simulink model "main_acs"  (R2025b)
settings: Solver=FixedStepAuto  StartTime=0.0  StopTime=20  FixedStep=0.001  RelTol=1e-3
values from neighbouring files (symbols this model uses):
  Actuator_MaxAngle = 8    [data.m]
  PID_Attitude_DCoeff_PY = 100    [data.m]
  PID_Attitude_DCoeff_R = 100    [data.m]
  PID_Attitude_Kd_PY = 0    [data.m]
  PID_Attitude_Kd_R = 0    [data.m]
  PID_Attitude_Ki_PY = 0    [data.m]
  PID_Attitude_Ki_R = 0    [data.m]
  PID_Attitude_Kp_PY = 2    [data.m]
  PID_Attitude_Kp_R = 2    [data.m]
  PID_Attitude_MaxOutput = 720    [data.m]
  PID_Attitude_SampleTime = 0.01    [data.m]
  PID_Guidance_K = 1/0.5    (= 2)    [data.m]
  PID_Guidance_MaxAcc = abs(5 * Physics_Gravity)    [data.m]
  PID_Guidance_N = 3.5    [data.m]
  PID_Guidance_SampleTime = 0.1    [data.m]
  PID_Rates_DCoeff_PY = 100    [data.m]
  PID_Rates_DCoeff_R = 100    [data.m]
  PID_Rates_Kd_PY = 0    [data.m]
  PID_Rates_Kd_R = 0    [data.m]
  PID_Rates_Ki_PY = 0    [data.m]
  PID_Rates_Ki_R = 0    [data.m]
  PID_Rates_Kp_PY = 400    [data.m]
  PID_Rates_Kp_R = 100    [data.m]
  PID_Rates_SampleTime = 0.002    [data.m]
libraries: slpidlib x6, simulink_extras x3, matrix_library x2, vrlib x1, aerolibanim x1
settings Model: Creator=Filip  LastModifiedBy=Filip
settings SolverCC: EnableFixedStepZeroCrossing=on
settings RTWCC: GenCodeOnly=on
settings SimscapeCC: SimscapeLogDecimation=1  SimscapeLogDataHistory=5000

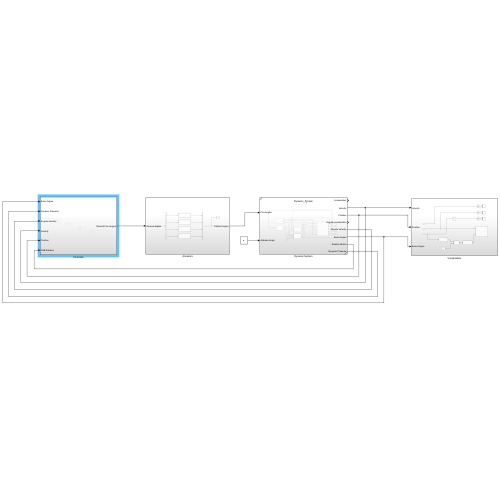
[thumbnail: Simulink's stored preview of the top-level diagram]
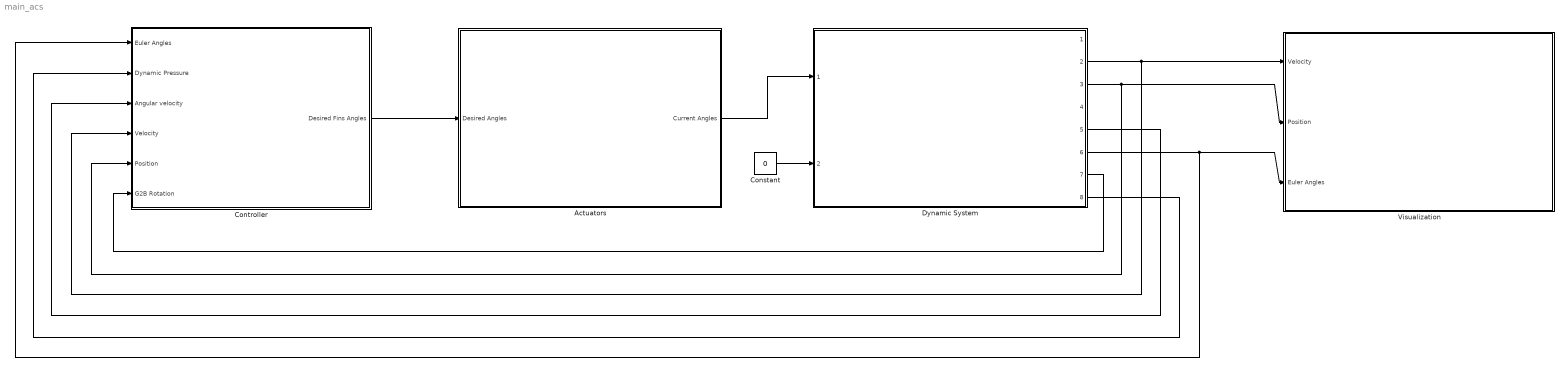
== system main_acs ==
  Actuators : Subsystem
  Constant : Constant  Value=0
  Controller : Subsystem
  Dynamic System : Subsystem  ReferencedSubsystem=Dynamic_System
  Visualization : Subsystem
  wires:
  Dynamic System/2 -> Controller/4(Velocity), Visualization/1(Velocity)
  Dynamic System/3 -> Controller/5(Position), Visualization/2(Position)
  Dynamic System/6 -> Controller/1(Euler Angles), Visualization/3(Euler Angles)
  Constant/1 -> Dynamic System/2
  Controller/1(Desired Fins Angles) -> Actuators/1(Desired Angles)
  Dynamic System/8 -> Controller/2(Dynamic Pressure)
  Dynamic System/5 -> Controller/3(Angular velocity)
  Dynamic System/7 -> Controller/6(G2B Rotation)
  Actuators/1(Current Angles) -> Dynamic System/1

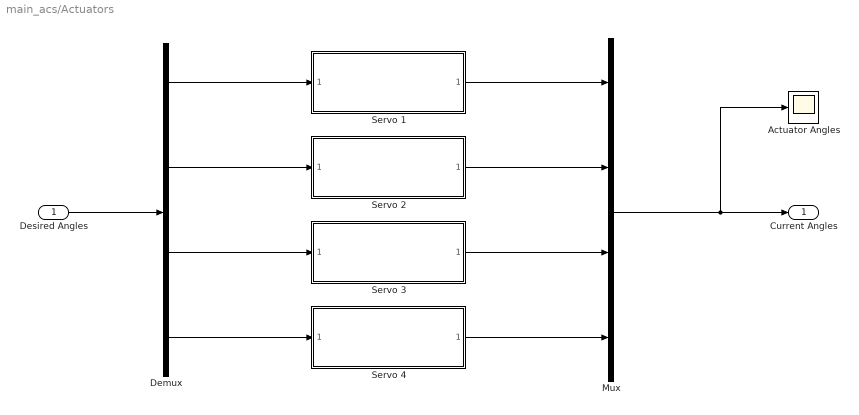
== system main_acs/Actuators ==
  Desired Angles : Inport
  Actuator Angles : Scope
      settings: ActiveDisplayYMinimum=-0.32568305206564774  ActiveDisplayYMaximum=0.47329758966714691  DataLoggingVariableName=ScopeData2
  Demux : Demux
  Mux : Mux
  Servo {1..4} (4 alike) : Subsystem  ReferencedSubsystem=Actuator_Dynamics
  Current Angles : Outport
  wires:
  Desired Angles/1 -> Demux/1
  Demux/1 -> Servo 1/1
  Demux/2 -> Servo 2/1
  Demux/3 -> Servo 3/1
  Demux/4 -> Servo 4/1
  Servo 1/1 -> Mux/1
  Servo 2/1 -> Mux/2
  Servo 3/1 -> Mux/3
  Servo 4/1 -> Mux/4
  Mux/1 -> Actuator Angles/1, Current Angles/1

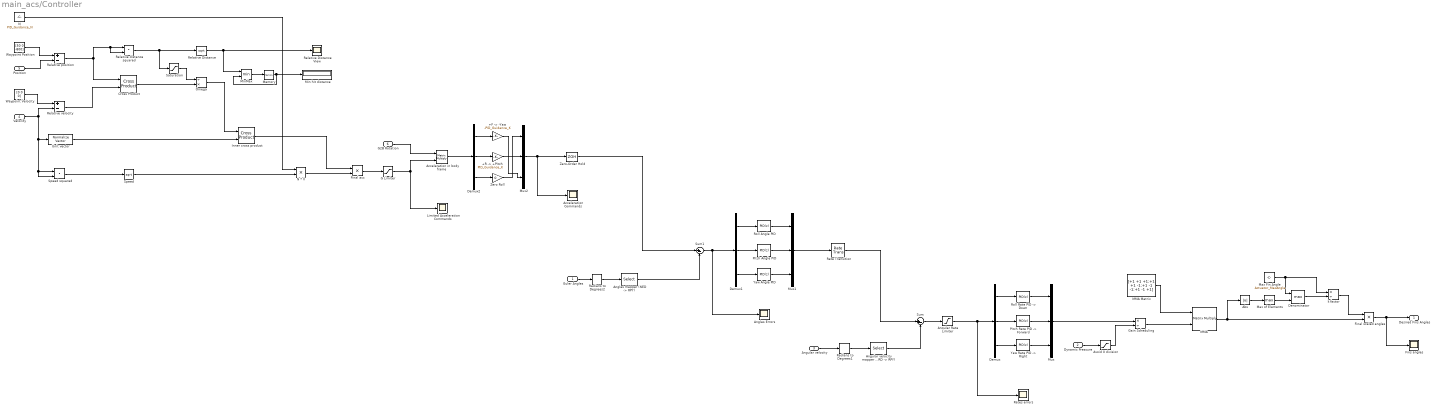
== system main_acs/Controller ==
  Euler Angles : Inport
  Dynamic Pressure : Inport  Port=2
  Angular velocity : Inport  Port=3
  Velocity : Inport  Port=4
  Position : Inport  Port=5
  G2B Rotation : Inport  Port=6
  "+F -> -Yaw" : Gain  Gain=-PID_Guidance_K
  "+R -> +Pitch" : Gain  Gain=PID_Guidance_K
  Abs : Abs  SaturateOnIntegerOverflow=off
  Acceleration Commands : Scope
      settings: ActiveDisplayYMinimum=-84.6659490201055  ActiveDisplayYMaximum=52.500724328147285  DataLoggingVariableName=ScopeData7
  Acceleration in body frame : Product  Multiplication=Matrix(*)
  Angles Errors : Scope
      settings: ActiveDisplayYMinimum=-272.55163687655789  ActiveDisplayYMaximum=253.11817045334493  DataLoggingVariableName=ScopeData6
  "Angles mapper (NED -> RPY)" : Selector  InputPortWidth=3  IndexOptions=Index vector (dialog)  Indices=[3 1 2]  OutputSizes=1
  Angular Rate Limiter : Saturate  UpperLimit=+PID_Attitude_MaxOutput  LowerLimit=-PID_Attitude_MaxOutput
  "Angular velocity mapper (FRD -> RPY)" : Selector  InputPortWidth=3  IndexOptions=Index vector (dialog)  Indices=[3 1 2]  OutputSizes=1
  Avoid 0 division : Saturate  UpperLimit=1000000  LowerLimit=10
  Cross Product : matrix_library/Cross Product
  Demux : Demux  Outputs=3
  Demux1 : Demux  Outputs=3
  Demux2 : Demux  Outputs=3
  Denominator : MinMax  Function=max  Inputs=2
  Final acc : Product
  Final scaled angles : Product
  Fins angles : Scope
      settings: ActiveDisplayYMinimum=-11.78731036094773  ActiveDisplayYMaximum=7.6919181875956841  DataLoggingVariableName=ScopeData5
  G Limiter : Saturate  UpperLimit=+PID_Guidance_MaxAcc  LowerLimit=-PID_Guidance_MaxAcc
  Gain Scheduling : Product  Inputs=*/
  Inner cross product : matrix_library/Cross Product
  Limited Acceleration Commands : Scope
      settings: ActiveDisplayYMinimum=-1  ActiveDisplayYMaximum=1  DataLoggingVariableName=ScopeData9
  MMA : Product  Multiplication=Matrix(*)
  MMA Matrix : Constant  Value=[+1 +1 +1;+1 +1 -1;+1 -1 -1;+1 -1 +1]
  Max Fin Angle : Constant  Value=Actuator_MaxAngle
  Max of Elements : MinMax  Function=max
  Memory : Memory  InitialCondition=inf
  Min hit distance : Display
  MinMax : MinMax  Inputs=2
  Mux : Mux  Inputs=3
  Mux1 : Mux  Inputs=3
  Mux2 : Mux  Inputs=3
  N : Constant  Value=PID_Guidance_N
  N * V : Product
  Omega : Product  Inputs=/*
  Pitch Angle PID : slpidlib/PID Controller  Controller=PID  Form=Parallel  TimeDomain=Discrete-time  UseExternalTs=off  SampleTime=PID_Attitude_SampleTime  IntegratorMethod=Forward Euler  FilterMethod=Forward Euler  ControllerParametersSource=internal  P=PID_Attitude_Kp_PY  I=PID_Attitude_Ki_PY  UseKiTs=off  D=PID_Attitude_Kd_PY  UseExternalDerivativeSource=off  N=PID_Attitude_DCoeff_PY  UseFilter=on  TunerSelectOption=Transfer Function Based (PID Tuner App)  InitialConditionSource=internal  InitialConditionForIntegrator=0  InitialConditionForFilter=0  DifferentiatorICPrevScaledInput=0  ExternalReset=none  TrackingMode=off  Kt=1  LimitOutput=off  SatLimitsSource=internal  UpperSaturationLimit=inf  LowerSaturationLimit=-inf  LinearizeAsGain=off  AntiWindupMode=back-calculation  Kb=1  LimitIntegrator=off  UpperIntegratorSaturationLimit=inf  LowerIntegratorSaturationLimit=-inf  POutMin=[]  POutMax=[]  IOutMin=[]  IOutMax=[]  DOutMin=[]  DOutMax=[]  NOutMin=[]  NOutMax=[]  SumOutMin=[]  SumOutMax=[]  SaturationOutMin=[]  SaturationOutMax=[]  PParamMin=[]  PParamMax=[]  IParamMin=[]  IParamMax=[]  DParamMin=[]  DParamMax=[]  NParamMin=[]  NParamMax=[]  KbParamMin=[]  KbParamMax=[]  KtParamMin=[]  KtParamMax=[]  KbOutMin=[]  KbOutMax=[]  KtOutMin=[]  KtOutMax=[]  IntegratorOutMin=[]  IntegratorOutMax=[]  FilterOutMin=[]  FilterOutMax=[]  SumI1OutMin=[]  SumI1OutMax=[]  SumI2OutMin=[]  SumI2OutMax=[]  SumI3OutMin=[]  SumI3OutMax=[]  SumI4OutMin=[]  SumI4OutMax=[]  SumDOutMin=[]  SumDOutMax=[]  DifferentiatorOutMin=[]  DifferentiatorOutMax=[]  FilterDiffOutCoefMin=[]  FilterDiffOutCoefMax=[]  ReciprocalOutMin=[]  ReciprocalOutMax=[]  SumDenOutMin=[]  SumDenOutMax=[]  SumNumOutMin=[]  SumNumOutMax=[]  DivideOutMin=[]  DivideOutMax=[]  UdiffTsProdOutMin=[]  UdiffTsProdOutMax=[]  NTsProdOutMin=[]  NTsProdOutMax=[]  UintegralTsProdOutMin=[]  UintegralTsProdOutMax=[]  UngainTsProdOutMin=[]  UngainTsProdOutMax=[]  ClampingZeroOutDataTypeStr=Inherit: Inherit via back propagation  ClampingZeroOutMin=[]  ClampingZeroOutMax=[]  FilterDenConstantOutDataTypeStr=Inherit: Inherit via back propagation  FilterDenConstantOutMin=[]  FilterDenConstantOutMax=[]  PCopyOutDataTypeStr=Inherit: Inherit via back propagation  PCopyOutMin=[]  PCopyOutMax=[]  NCopyOutDataTypeStr=Inherit: Inherit via back propagation  NCopyOutMin=[]  NCopyOutMax=[]  IntegratorContinuousStateAttributes=''  IntegratorStateMustResolveToSignalObject=off  IntegratorRTWStateStorageClass=Auto  FilterContinuousStateAttributes=''  FilterStateMustResolveToSignalObject=off  FilterRTWStateStorageClass=Auto  ParallelPVariant=InternalParameters  IdealPVariant=Disabled  IVariant=InternalParameters  DVariant=InternalParameters  IntegratorVariant=Discrete  SatVariant=Disabled  AWVariant=Passthrough  PCopyVariant=Disabled  TRVariant=Disabled  FdbkBlocksVariant=Forward  IdealPFdbkVariant=Disabled  SatFdbkVariant=Disabled  DerivativeFilterVariant=ForwardEulerFilter  NVariant=InternalParameters  NCopyVariant=Disabled  FilterICVariant=InternalICsFilter  IntegratorICVariant=InternalICs  ExternalResetVariant=Disabled  TRSumVariant=Passthrough  SumFdbkVariant=Disabled  SumVariant=Sum_PID  TsampFilterVariant=InternalTs  TsampNgainVariant=Passthrough  TsampIntegralVariant=Disabled_SignalSpec  ExternalSaturationOutDataTypeStr=Inherit: Same as second input  DerivativeSourceVariant=ErrorSignal  PreIntVariant=InternalPreInt
      settings: LibrarySourceBlock=simulink/Discrete/Discrete PID Controller
  "Pitch Rate PID -> Forward" : slpidlib/PID Controller  Controller=PID  Form=Parallel  TimeDomain=Discrete-time  UseExternalTs=off  SampleTime=PID_Rates_SampleTime  IntegratorMethod=Forward Euler  FilterMethod=Forward Euler  ControllerParametersSource=internal  P=PID_Rates_Kp_PY  I=PID_Rates_Ki_PY  UseKiTs=off  D=PID_Rates_Kd_PY  UseExternalDerivativeSource=off  N=PID_Rates_DCoeff_PY  UseFilter=on  TunerSelectOption=Transfer Function Based (PID Tuner App)  InitialConditionSource=internal  InitialConditionForIntegrator=0  InitialConditionForFilter=0  DifferentiatorICPrevScaledInput=0  ExternalReset=none  TrackingMode=off  Kt=1  LimitOutput=off  SatLimitsSource=internal  UpperSaturationLimit=inf  LowerSaturationLimit=-inf  LinearizeAsGain=off  AntiWindupMode=back-calculation  Kb=1  LimitIntegrator=off  UpperIntegratorSaturationLimit=inf  LowerIntegratorSaturationLimit=-inf  POutMin=[]  POutMax=[]  IOutMin=[]  IOutMax=[]  DOutMin=[]  DOutMax=[]  NOutMin=[]  NOutMax=[]  SumOutMin=[]  SumOutMax=[]  SaturationOutMin=[]  SaturationOutMax=[]  PParamMin=[]  PParamMax=[]  IParamMin=[]  IParamMax=[]  DParamMin=[]  DParamMax=[]  NParamMin=[]  NParamMax=[]  KbParamMin=[]  KbParamMax=[]  KtParamMin=[]  KtParamMax=[]  KbOutMin=[]  KbOutMax=[]  KtOutMin=[]  KtOutMax=[]  IntegratorOutMin=[]  IntegratorOutMax=[]  FilterOutMin=[]  FilterOutMax=[]  SumI1OutMin=[]  SumI1OutMax=[]  SumI2OutMin=[]  SumI2OutMax=[]  SumI3OutMin=[]  SumI3OutMax=[]  SumI4OutMin=[]  SumI4OutMax=[]  SumDOutMin=[]  SumDOutMax=[]  DifferentiatorOutMin=[]  DifferentiatorOutMax=[]  FilterDiffOutCoefMin=[]  FilterDiffOutCoefMax=[]  ReciprocalOutMin=[]  ReciprocalOutMax=[]  SumDenOutMin=[]  SumDenOutMax=[]  SumNumOutMin=[]  SumNumOutMax=[]  DivideOutMin=[]  DivideOutMax=[]  UdiffTsProdOutMin=[]  UdiffTsProdOutMax=[]  NTsProdOutMin=[]  NTsProdOutMax=[]  UintegralTsProdOutMin=[]  UintegralTsProdOutMax=[]  UngainTsProdOutMin=[]  UngainTsProdOutMax=[]  ClampingZeroOutDataTypeStr=Inherit: Inherit via back propagation  ClampingZeroOutMin=[]  ClampingZeroOutMax=[]  FilterDenConstantOutDataTypeStr=Inherit: Inherit via back propagation  FilterDenConstantOutMin=[]  FilterDenConstantOutMax=[]  PCopyOutDataTypeStr=Inherit: Inherit via back propagation  PCopyOutMin=[]  PCopyOutMax=[]  NCopyOutDataTypeStr=Inherit: Inherit via back propagation  NCopyOutMin=[]  NCopyOutMax=[]  IntegratorContinuousStateAttributes=''  IntegratorStateMustResolveToSignalObject=off  IntegratorRTWStateStorageClass=Auto  FilterContinuousStateAttributes=''  FilterStateMustResolveToSignalObject=off  FilterRTWStateStorageClass=Auto  ParallelPVariant=InternalParameters  IdealPVariant=Disabled  IVariant=InternalParameters  DVariant=InternalParameters  IntegratorVariant=Discrete  SatVariant=Disabled  AWVariant=Passthrough  PCopyVariant=Disabled  TRVariant=Disabled  FdbkBlocksVariant=Forward  IdealPFdbkVariant=Disabled  SatFdbkVariant=Disabled  DerivativeFilterVariant=ForwardEulerFilter  NVariant=InternalParameters  NCopyVariant=Disabled  FilterICVariant=InternalICsFilter  IntegratorICVariant=InternalICs  ExternalResetVariant=Disabled  TRSumVariant=Passthrough  SumFdbkVariant=Disabled  SumVariant=Sum_PID  TsampFilterVariant=InternalTs  TsampNgainVariant=Passthrough  TsampIntegralVariant=Disabled_SignalSpec  ExternalSaturationOutDataTypeStr=Inherit: Same as second input  DerivativeSourceVariant=ErrorSignal  PreIntVariant=InternalPreInt
      settings: LibrarySourceBlock=simulink/Discrete/Discrete PID Controller
  Radians to Degrees1 : simulink_extras/Transformations/Radians to Degrees
  Radians to Degrees2 : simulink_extras/Transformations/Radians to Degrees
  Rate Transition : RateTransition
  Rates errors : Scope
      settings: ActiveDisplayYMinimum=-72.348500996231849  ActiveDisplayYMaximum=106.71571719199865  DataLoggingVariableName=ScopeData4
  Relative Distance : Sqrt
  Relative Distance View : Scope
      settings: ActiveDisplayYMinimum=-3326.7909111536519  ActiveDisplayYMaximum=1807.9538182461531  DataLoggingVariableName=ScopeData8
  Relative distance squared : DotProduct  OutDataTypeStr=Inherit: Inherit via internal rule
  Relative position : Sum  Inputs=+-
  Relative velocity : Sum  Inputs=+-
  Roll Angle PID : slpidlib/PID Controller  Controller=PID  Form=Parallel  TimeDomain=Discrete-time  UseExternalTs=off  SampleTime=PID_Attitude_SampleTime  IntegratorMethod=Forward Euler  FilterMethod=Forward Euler  ControllerParametersSource=internal  P=PID_Attitude_Kp_R  I=PID_Attitude_Ki_R  UseKiTs=off  D=PID_Attitude_Kd_R  UseExternalDerivativeSource=off  N=PID_Attitude_DCoeff_R  UseFilter=on  TunerSelectOption=Transfer Function Based (PID Tuner App)  InitialConditionSource=internal  InitialConditionForIntegrator=0  InitialConditionForFilter=0  DifferentiatorICPrevScaledInput=0  ExternalReset=none  TrackingMode=off  Kt=1  LimitOutput=off  SatLimitsSource=internal  UpperSaturationLimit=inf  LowerSaturationLimit=-inf  LinearizeAsGain=off  AntiWindupMode=back-calculation  Kb=1  LimitIntegrator=off  UpperIntegratorSaturationLimit=inf  LowerIntegratorSaturationLimit=-inf  POutMin=[]  POutMax=[]  IOutMin=[]  IOutMax=[]  DOutMin=[]  DOutMax=[]  NOutMin=[]  NOutMax=[]  SumOutMin=[]  SumOutMax=[]  SaturationOutMin=[]  SaturationOutMax=[]  PParamMin=[]  PParamMax=[]  IParamMin=[]  IParamMax=[]  DParamMin=[]  DParamMax=[]  NParamMin=[]  NParamMax=[]  KbParamMin=[]  KbParamMax=[]  KtParamMin=[]  KtParamMax=[]  KbOutMin=[]  KbOutMax=[]  KtOutMin=[]  KtOutMax=[]  IntegratorOutMin=[]  IntegratorOutMax=[]  FilterOutMin=[]  FilterOutMax=[]  SumI1OutMin=[]  SumI1OutMax=[]  SumI2OutMin=[]  SumI2OutMax=[]  SumI3OutMin=[]  SumI3OutMax=[]  SumI4OutMin=[]  SumI4OutMax=[]  SumDOutMin=[]  SumDOutMax=[]  DifferentiatorOutMin=[]  DifferentiatorOutMax=[]  FilterDiffOutCoefMin=[]  FilterDiffOutCoefMax=[]  ReciprocalOutMin=[]  ReciprocalOutMax=[]  SumDenOutMin=[]  SumDenOutMax=[]  SumNumOutMin=[]  SumNumOutMax=[]  DivideOutMin=[]  DivideOutMax=[]  UdiffTsProdOutMin=[]  UdiffTsProdOutMax=[]  NTsProdOutMin=[]  NTsProdOutMax=[]  UintegralTsProdOutMin=[]  UintegralTsProdOutMax=[]  UngainTsProdOutMin=[]  UngainTsProdOutMax=[]  ClampingZeroOutDataTypeStr=Inherit: Inherit via back propagation  ClampingZeroOutMin=[]  ClampingZeroOutMax=[]  FilterDenConstantOutDataTypeStr=Inherit: Inherit via back propagation  FilterDenConstantOutMin=[]  FilterDenConstantOutMax=[]  PCopyOutDataTypeStr=Inherit: Inherit via back propagation  PCopyOutMin=[]  PCopyOutMax=[]  NCopyOutDataTypeStr=Inherit: Inherit via back propagation  NCopyOutMin=[]  NCopyOutMax=[]  IntegratorContinuousStateAttributes=''  IntegratorStateMustResolveToSignalObject=off  IntegratorRTWStateStorageClass=Auto  FilterContinuousStateAttributes=''  FilterStateMustResolveToSignalObject=off  FilterRTWStateStorageClass=Auto  ParallelPVariant=InternalParameters  IdealPVariant=Disabled  IVariant=InternalParameters  DVariant=InternalParameters  IntegratorVariant=Discrete  SatVariant=Disabled  AWVariant=Passthrough  PCopyVariant=Disabled  TRVariant=Disabled  FdbkBlocksVariant=Forward  IdealPFdbkVariant=Disabled  SatFdbkVariant=Disabled  DerivativeFilterVariant=ForwardEulerFilter  NVariant=InternalParameters  NCopyVariant=Disabled  FilterICVariant=InternalICsFilter  IntegratorICVariant=InternalICs  ExternalResetVariant=Disabled  TRSumVariant=Passthrough  SumFdbkVariant=Disabled  SumVariant=Sum_PID  TsampFilterVariant=InternalTs  TsampNgainVariant=Passthrough  TsampIntegralVariant=Disabled_SignalSpec  ExternalSaturationOutDataTypeStr=Inherit: Same as second input  DerivativeSourceVariant=ErrorSignal  PreIntVariant=InternalPreInt
      settings: LibrarySourceBlock=simulink/Discrete/Discrete PID Controller
  "Roll Rate PID -> Down" : slpidlib/PID Controller  Controller=PID  Form=Parallel  TimeDomain=Discrete-time  UseExternalTs=off  SampleTime=PID_Rates_SampleTime  IntegratorMethod=Forward Euler  FilterMethod=Forward Euler  ControllerParametersSource=internal  P=PID_Rates_Kp_R  I=PID_Rates_Ki_R  UseKiTs=off  D=PID_Rates_Kd_R  UseExternalDerivativeSource=off  N=PID_Rates_DCoeff_R  UseFilter=on  TunerSelectOption=Transfer Function Based (PID Tuner App)  InitialConditionSource=internal  InitialConditionForIntegrator=0  InitialConditionForFilter=0  DifferentiatorICPrevScaledInput=0  ExternalReset=none  TrackingMode=off  Kt=1  LimitOutput=off  SatLimitsSource=internal  UpperSaturationLimit=inf  LowerSaturationLimit=-inf  LinearizeAsGain=off  AntiWindupMode=back-calculation  Kb=1  LimitIntegrator=off  UpperIntegratorSaturationLimit=inf  LowerIntegratorSaturationLimit=-inf  POutMin=[]  POutMax=[]  IOutMin=[]  IOutMax=[]  DOutMin=[]  DOutMax=[]  NOutMin=[]  NOutMax=[]  SumOutMin=[]  SumOutMax=[]  SaturationOutMin=[]  SaturationOutMax=[]  PParamMin=[]  PParamMax=[]  IParamMin=[]  IParamMax=[]  DParamMin=[]  DParamMax=[]  NParamMin=[]  NParamMax=[]  KbParamMin=[]  KbParamMax=[]  KtParamMin=[]  KtParamMax=[]  KbOutMin=[]  KbOutMax=[]  KtOutMin=[]  KtOutMax=[]  IntegratorOutMin=[]  IntegratorOutMax=[]  FilterOutMin=[]  FilterOutMax=[]  SumI1OutMin=[]  SumI1OutMax=[]  SumI2OutMin=[]  SumI2OutMax=[]  SumI3OutMin=[]  SumI3OutMax=[]  SumI4OutMin=[]  SumI4OutMax=[]  SumDOutMin=[]  SumDOutMax=[]  DifferentiatorOutMin=[]  DifferentiatorOutMax=[]  FilterDiffOutCoefMin=[]  FilterDiffOutCoefMax=[]  ReciprocalOutMin=[]  ReciprocalOutMax=[]  SumDenOutMin=[]  SumDenOutMax=[]  SumNumOutMin=[]  SumNumOutMax=[]  DivideOutMin=[]  DivideOutMax=[]  UdiffTsProdOutMin=[]  UdiffTsProdOutMax=[]  NTsProdOutMin=[]  NTsProdOutMax=[]  UintegralTsProdOutMin=[]  UintegralTsProdOutMax=[]  UngainTsProdOutMin=[]  UngainTsProdOutMax=[]  ClampingZeroOutDataTypeStr=Inherit: Inherit via back propagation  ClampingZeroOutMin=[]  ClampingZeroOutMax=[]  FilterDenConstantOutDataTypeStr=Inherit: Inherit via back propagation  FilterDenConstantOutMin=[]  FilterDenConstantOutMax=[]  PCopyOutDataTypeStr=Inherit: Inherit via back propagation  PCopyOutMin=[]  PCopyOutMax=[]  NCopyOutDataTypeStr=Inherit: Inherit via back propagation  NCopyOutMin=[]  NCopyOutMax=[]  IntegratorContinuousStateAttributes=''  IntegratorStateMustResolveToSignalObject=off  IntegratorRTWStateStorageClass=Auto  FilterContinuousStateAttributes=''  FilterStateMustResolveToSignalObject=off  FilterRTWStateStorageClass=Auto  ParallelPVariant=InternalParameters  IdealPVariant=Disabled  IVariant=InternalParameters  DVariant=InternalParameters  IntegratorVariant=Discrete  SatVariant=Disabled  AWVariant=Passthrough  PCopyVariant=Disabled  TRVariant=Disabled  FdbkBlocksVariant=Forward  IdealPFdbkVariant=Disabled  SatFdbkVariant=Disabled  DerivativeFilterVariant=ForwardEulerFilter  NVariant=InternalParameters  NCopyVariant=Disabled  FilterICVariant=InternalICsFilter  IntegratorICVariant=InternalICs  ExternalResetVariant=Disabled  TRSumVariant=Passthrough  SumFdbkVariant=Disabled  SumVariant=Sum_PID  TsampFilterVariant=InternalTs  TsampNgainVariant=Passthrough  TsampIntegralVariant=Disabled_SignalSpec  ExternalSaturationOutDataTypeStr=Inherit: Same as second input  DerivativeSourceVariant=ErrorSignal  PreIntVariant=InternalPreInt
      settings: LibrarySourceBlock=simulink/Discrete/Discrete PID Controller
  Saturation : Saturate  UpperLimit=10000000  LowerLimit=400
  Speed : Sqrt
  Speed squared : DotProduct  OutDataTypeStr=Inherit: Inherit via internal rule
  Sum : Sum  Inputs=|+-
  Sum1 : Sum  Inputs=|+-
  Unit vector : vrlib/Utilities/Normalize Vector  maxzero=0
  Waypoint Position : Constant  Value=[50 0 -800]
  Waypoint Velocity : Constant  Value=[0 0 0]
  Yaw Angle PID : slpidlib/PID Controller  Controller=PID  Form=Parallel  TimeDomain=Discrete-time  UseExternalTs=off  SampleTime=PID_Attitude_SampleTime  IntegratorMethod=Forward Euler  FilterMethod=Forward Euler  ControllerParametersSource=internal  P=PID_Attitude_Kp_PY  I=PID_Attitude_Ki_PY  UseKiTs=off  D=PID_Attitude_Kd_PY  UseExternalDerivativeSource=off  N=PID_Attitude_DCoeff_PY  UseFilter=on  TunerSelectOption=Transfer Function Based (PID Tuner App)  InitialConditionSource=internal  InitialConditionForIntegrator=0  InitialConditionForFilter=0  DifferentiatorICPrevScaledInput=0  ExternalReset=none  TrackingMode=off  Kt=1  LimitOutput=off  SatLimitsSource=internal  UpperSaturationLimit=inf  LowerSaturationLimit=-inf  LinearizeAsGain=off  AntiWindupMode=back-calculation  Kb=1  LimitIntegrator=off  UpperIntegratorSaturationLimit=inf  LowerIntegratorSaturationLimit=-inf  POutMin=[]  POutMax=[]  IOutMin=[]  IOutMax=[]  DOutMin=[]  DOutMax=[]  NOutMin=[]  NOutMax=[]  SumOutMin=[]  SumOutMax=[]  SaturationOutMin=[]  SaturationOutMax=[]  PParamMin=[]  PParamMax=[]  IParamMin=[]  IParamMax=[]  DParamMin=[]  DParamMax=[]  NParamMin=[]  NParamMax=[]  KbParamMin=[]  KbParamMax=[]  KtParamMin=[]  KtParamMax=[]  KbOutMin=[]  KbOutMax=[]  KtOutMin=[]  KtOutMax=[]  IntegratorOutMin=[]  IntegratorOutMax=[]  FilterOutMin=[]  FilterOutMax=[]  SumI1OutMin=[]  SumI1OutMax=[]  SumI2OutMin=[]  SumI2OutMax=[]  SumI3OutMin=[]  SumI3OutMax=[]  SumI4OutMin=[]  SumI4OutMax=[]  SumDOutMin=[]  SumDOutMax=[]  DifferentiatorOutMin=[]  DifferentiatorOutMax=[]  FilterDiffOutCoefMin=[]  FilterDiffOutCoefMax=[]  ReciprocalOutMin=[]  ReciprocalOutMax=[]  SumDenOutMin=[]  SumDenOutMax=[]  SumNumOutMin=[]  SumNumOutMax=[]  DivideOutMin=[]  DivideOutMax=[]  UdiffTsProdOutMin=[]  UdiffTsProdOutMax=[]  NTsProdOutMin=[]  NTsProdOutMax=[]  UintegralTsProdOutMin=[]  UintegralTsProdOutMax=[]  UngainTsProdOutMin=[]  UngainTsProdOutMax=[]  ClampingZeroOutDataTypeStr=Inherit: Inherit via back propagation  ClampingZeroOutMin=[]  ClampingZeroOutMax=[]  FilterDenConstantOutDataTypeStr=Inherit: Inherit via back propagation  FilterDenConstantOutMin=[]  FilterDenConstantOutMax=[]  PCopyOutDataTypeStr=Inherit: Inherit via back propagation  PCopyOutMin=[]  PCopyOutMax=[]  NCopyOutDataTypeStr=Inherit: Inherit via back propagation  NCopyOutMin=[]  NCopyOutMax=[]  IntegratorContinuousStateAttributes=''  IntegratorStateMustResolveToSignalObject=off  IntegratorRTWStateStorageClass=Auto  FilterContinuousStateAttributes=''  FilterStateMustResolveToSignalObject=off  FilterRTWStateStorageClass=Auto  ParallelPVariant=InternalParameters  IdealPVariant=Disabled  IVariant=InternalParameters  DVariant=InternalParameters  IntegratorVariant=Discrete  SatVariant=Disabled  AWVariant=Passthrough  PCopyVariant=Disabled  TRVariant=Disabled  FdbkBlocksVariant=Forward  IdealPFdbkVariant=Disabled  SatFdbkVariant=Disabled  DerivativeFilterVariant=ForwardEulerFilter  NVariant=InternalParameters  NCopyVariant=Disabled  FilterICVariant=InternalICsFilter  IntegratorICVariant=InternalICs  ExternalResetVariant=Disabled  TRSumVariant=Passthrough  SumFdbkVariant=Disabled  SumVariant=Sum_PID  TsampFilterVariant=InternalTs  TsampNgainVariant=Passthrough  TsampIntegralVariant=Disabled_SignalSpec  ExternalSaturationOutDataTypeStr=Inherit: Same as second input  DerivativeSourceVariant=ErrorSignal  PreIntVariant=InternalPreInt
      settings: LibrarySourceBlock=simulink/Discrete/Discrete PID Controller
  "Yaw Rate PID -> Right" : slpidlib/PID Controller  Controller=PID  Form=Parallel  TimeDomain=Discrete-time  UseExternalTs=off  SampleTime=PID_Rates_SampleTime  IntegratorMethod=Forward Euler  FilterMethod=Forward Euler  ControllerParametersSource=internal  P=PID_Rates_Kp_PY  I=PID_Rates_Ki_PY  UseKiTs=off  D=PID_Rates_Kd_PY  UseExternalDerivativeSource=off  N=PID_Rates_DCoeff_PY  UseFilter=on  TunerSelectOption=Transfer Function Based (PID Tuner App)  InitialConditionSource=internal  InitialConditionForIntegrator=0  InitialConditionForFilter=0  DifferentiatorICPrevScaledInput=0  ExternalReset=none  TrackingMode=off  Kt=1  LimitOutput=off  SatLimitsSource=internal  UpperSaturationLimit=inf  LowerSaturationLimit=-inf  LinearizeAsGain=off  AntiWindupMode=back-calculation  Kb=1  LimitIntegrator=off  UpperIntegratorSaturationLimit=inf  LowerIntegratorSaturationLimit=-inf  POutMin=[]  POutMax=[]  IOutMin=[]  IOutMax=[]  DOutMin=[]  DOutMax=[]  NOutMin=[]  NOutMax=[]  SumOutMin=[]  SumOutMax=[]  SaturationOutMin=[]  SaturationOutMax=[]  PParamMin=[]  PParamMax=[]  IParamMin=[]  IParamMax=[]  DParamMin=[]  DParamMax=[]  NParamMin=[]  NParamMax=[]  KbParamMin=[]  KbParamMax=[]  KtParamMin=[]  KtParamMax=[]  KbOutMin=[]  KbOutMax=[]  KtOutMin=[]  KtOutMax=[]  IntegratorOutMin=[]  IntegratorOutMax=[]  FilterOutMin=[]  FilterOutMax=[]  SumI1OutMin=[]  SumI1OutMax=[]  SumI2OutMin=[]  SumI2OutMax=[]  SumI3OutMin=[]  SumI3OutMax=[]  SumI4OutMin=[]  SumI4OutMax=[]  SumDOutMin=[]  SumDOutMax=[]  DifferentiatorOutMin=[]  DifferentiatorOutMax=[]  FilterDiffOutCoefMin=[]  FilterDiffOutCoefMax=[]  ReciprocalOutMin=[]  ReciprocalOutMax=[]  SumDenOutMin=[]  SumDenOutMax=[]  SumNumOutMin=[]  SumNumOutMax=[]  DivideOutMin=[]  DivideOutMax=[]  UdiffTsProdOutMin=[]  UdiffTsProdOutMax=[]  NTsProdOutMin=[]  NTsProdOutMax=[]  UintegralTsProdOutMin=[]  UintegralTsProdOutMax=[]  UngainTsProdOutMin=[]  UngainTsProdOutMax=[]  ClampingZeroOutDataTypeStr=Inherit: Inherit via back propagation  ClampingZeroOutMin=[]  ClampingZeroOutMax=[]  FilterDenConstantOutDataTypeStr=Inherit: Inherit via back propagation  FilterDenConstantOutMin=[]  FilterDenConstantOutMax=[]  PCopyOutDataTypeStr=Inherit: Inherit via back propagation  PCopyOutMin=[]  PCopyOutMax=[]  NCopyOutDataTypeStr=Inherit: Inherit via back propagation  NCopyOutMin=[]  NCopyOutMax=[]  IntegratorContinuousStateAttributes=''  IntegratorStateMustResolveToSignalObject=off  IntegratorRTWStateStorageClass=Auto  FilterContinuousStateAttributes=''  FilterStateMustResolveToSignalObject=off  FilterRTWStateStorageClass=Auto  ParallelPVariant=InternalParameters  IdealPVariant=Disabled  IVariant=InternalParameters  DVariant=InternalParameters  IntegratorVariant=Discrete  SatVariant=Disabled  AWVariant=Passthrough  PCopyVariant=Disabled  TRVariant=Disabled  FdbkBlocksVariant=Forward  IdealPFdbkVariant=Disabled  SatFdbkVariant=Disabled  DerivativeFilterVariant=ForwardEulerFilter  NVariant=InternalParameters  NCopyVariant=Disabled  FilterICVariant=InternalICsFilter  IntegratorICVariant=InternalICs  ExternalResetVariant=Disabled  TRSumVariant=Passthrough  SumFdbkVariant=Disabled  SumVariant=Sum_PID  TsampFilterVariant=InternalTs  TsampNgainVariant=Passthrough  TsampIntegralVariant=Disabled_SignalSpec  ExternalSaturationOutDataTypeStr=Inherit: Same as second input  DerivativeSourceVariant=ErrorSignal  PreIntVariant=InternalPreInt
      settings: LibrarySourceBlock=simulink/Discrete/Discrete PID Controller
  Zero Roll : Gain  Gain=0
  Zero-Order Hold : ZeroOrderHold  SampleTime=PID_Guidance_SampleTime
  k factor : Product  Inputs=*/
  Desired Fins Angles : Outport
  wires:
  Dynamic Pressure/1 -> Avoid 0 division/1
  Demux/1 -> "Roll Rate PID -> Down"/1
  Demux/2 -> "Pitch Rate PID -> Forward"/1
  Demux/3 -> "Yaw Rate PID -> Right"/1
  "Pitch Rate PID -> Forward"/1 -> Mux/2
  "Roll Rate PID -> Down"/1 -> Mux/1
  "Yaw Rate PID -> Right"/1 -> Mux/3
  MMA Matrix/1 -> MMA/1
  MMA/1 -> Final scaled angles/2, Abs/1
  Abs/1 -> Max of Elements/1
  Mux/1 -> Gain Scheduling/1
  Avoid 0 division/1 -> Gain Scheduling/2
  Gain Scheduling/1 -> MMA/2
  Radians to Degrees1/1 -> "Angular velocity mapper (FRD -> RPY)"/1
  Max of Elements/1 -> Denominator/2
  Max Fin Angle/1 -> Denominator/1, k factor/1
  Denominator/1 -> k factor/2
  Final scaled angles/1 -> Desired Fins Angles/1, Fins angles/1
  k factor/1 -> Final scaled angles/1
  Radians to Degrees2/1 -> "Angles mapper (NED -> RPY)"/1
  Pitch Angle PID/1 -> Mux1/2
  Demux1/3 -> Yaw Angle PID/1
  Demux1/2 -> Pitch Angle PID/1
  Demux1/1 -> Roll Angle PID/1
  Sum1/1 -> Demux1/1, Angles Errors/1
  Roll Angle PID/1 -> Mux1/1
  Yaw Angle PID/1 -> Mux1/3
  Mux1/1 -> Rate Transition/1
  Sum/1 -> Angular Rate Limiter/1
  Angular Rate Limiter/1 -> Rates errors/1, Demux/1
  Angular velocity/1 -> Radians to Degrees1/1
  "Angular velocity mapper (FRD -> RPY)"/1 -> Sum/2
  Euler Angles/1 -> Radians to Degrees2/1
  "Angles mapper (NED -> RPY)"/1 -> Sum1/2
  Velocity/1 -> Relative velocity/2, Speed squared/2, Speed squared/1, Unit vector/1
  Waypoint Position/1 -> Relative position/1
  Position/1 -> Relative position/2
  Waypoint Velocity/1 -> Relative velocity/1
  Relative position/1 -> Relative distance squared/2, Relative distance squared/1, Cross Product/1
  Relative velocity/1 -> Cross Product/2
  Cross Product/1 -> Omega/2
  Omega/1 -> Inner cross product/1
  Unit vector/1 -> Inner cross product/2
  N/1 -> N * V/1
  N * V/1 -> Final acc/2
  Inner cross product/1 -> Final acc/1
  Relative distance squared/1 -> Saturation/1, Relative Distance/1
  Speed squared/1 -> Speed/1
  Speed/1 -> N * V/2
  Relative Distance/1 -> MinMax/1, Relative Distance View/1
  Final acc/1 -> G Limiter/1
  G Limiter/1 -> Limited Acceleration Commands/1, Acceleration in body frame/2
  G2B Rotation/1 -> Acceleration in body frame/1
  Acceleration in body frame/1 -> Demux2/1
  Demux2/1 -> "+F -> -Yaw"/1
  Demux2/2 -> "+R -> +Pitch"/1
  Demux2/3 -> Zero Roll/1
  Mux2/1 -> Acceleration Commands/1, Zero-Order Hold/1
  Zero Roll/1 -> Mux2/1
  "+F -> -Yaw"/1 -> Mux2/3
  "+R -> +Pitch"/1 -> Mux2/2
  MinMax/1 -> Memory/1
  Memory/1 -> MinMax/2, Min hit distance/1
  Rate Transition/1 -> Sum/1
  Zero-Order Hold/1 -> Sum1/1
  Saturation/1 -> Omega/1

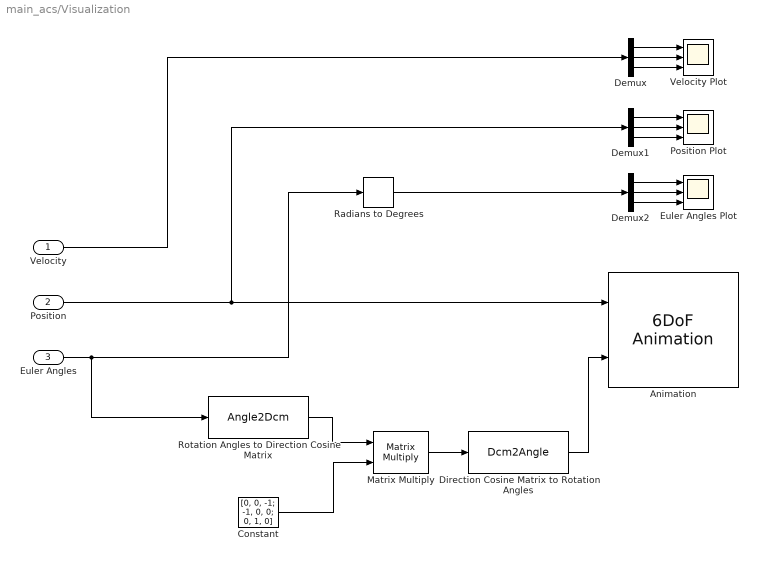
== system main_acs/Visualization ==
  Velocity : Inport
  Position : Inport  Port=2
  Euler Angles : Inport  Port=3
  Animation : aerolibanim/6DoF Animation  u1=[-4000 4000 -4000 4000 -4000 4000]  u2=0.01  u3=5  u4=[0 0 10]  u5=Fly alongside  u6=[-100 0 -50]  u7=10  u8=off
  Constant : Constant  Value=[0, 0, -1; -1, 0, 0; 0, 1, 0]  VectorParams1D=off
  Demux : Demux  Outputs=3
  Demux1 : Demux  Outputs=3
  Demux2 : Demux  Outputs=3
  Direction Cosine Matrix to Rotation Angles : Dcm2Angle
      settings: AttributesFormatString=Rotation Order: %<rotationOrder>
  Euler Angles Plot : Scope  NumInputPorts=3
      settings: ActiveDisplayYMinimum=-207.66502545433633  ActiveDisplayYMaximum=242.23354829591378  DataLoggingVariableName=ScopeData2
  Matrix Multiply : Product  Multiplication=Matrix(*)
  Position Plot : Scope  NumInputPorts=3
      settings: ActiveDisplayYMinimum=154.90803392721904  ActiveDisplayYMaximum=1200.6231108644074
  Radians to Degrees : simulink_extras/Transformations/Radians to Degrees
  Rotation Angles to Direction Cosine Matrix : Angle2Dcm
      settings: AttributesFormatString=Rotation Order: %<rotationOrder>
  Velocity Plot : Scope  NumInputPorts=3
      settings: ActiveDisplayYMinimum=-1  ActiveDisplayYMaximum=1
  wires:
  Demux1/2 -> Position Plot/2
  Demux2/1 -> Euler Angles Plot/1
  Demux1/3 -> Position Plot/3
  Demux/2 -> Velocity Plot/2
  Demux1/1 -> Position Plot/1
  Demux/3 -> Velocity Plot/3
  Demux/1 -> Velocity Plot/1
  Demux2/2 -> Euler Angles Plot/2
  Demux2/3 -> Euler Angles Plot/3
  Velocity/1 -> Demux/1
  Radians to Degrees/1 -> Demux2/1
  Position/1 -> Animation/1, Demux1/1
  Euler Angles/1 -> Rotation Angles to Direction Cosine Matrix/1, Radians to Degrees/1
  Matrix Multiply/1 -> Direction Cosine Matrix to Rotation Angles/1
  Direction Cosine Matrix to Rotation Angles/1 -> Animation/2
  Rotation Angles to Direction Cosine Matrix/1 -> Matrix Multiply/1
  Constant/1 -> Matrix Multiply/2
